simulink model "Lecture16_LSFIntegrator"  (R2020b)
settings: Solver=VariableStepAuto  StartTime=0.0  StopTime=10  RelTol=1e-3
values from neighbouring files (symbols this model uses):
  A = [0 1; -5 -2]    [Assignment4.m]    (also in Lecture14_LSF.m = [0 1; -1 -2]; Lecture15_DigitalLSF.m = [0 1; -1 -2]; Lecture16_LSFIntegrator.m = [0 1; -1 -2]; Lecture6_3PhaseCurrent.m = 20)
  B = [0; 1]    [Assignment4.m]    (also in Lecture14_LSF.m; Lecture15_DigitalLSF.m; Lecture16_LSFIntegrator.m; dSpaceLab.m = [0; 1/La])
  C = [5 0]    [Assignment4.m]    (also in Lecture14_LSF.m = [10 0]; Lecture15_DigitalLSF.m = [10 0]; Lecture16_LSFIntegrator.m = [10 0]; dSpaceLab.m = [1, 0])
  K12 = [K(1) K(2)]    [Assignment4.m]    (also in Lecture16_LSFIntegrator.m)
  Ki = 1/2    (= 0.5)    [Assignment3.m]    (also in Assignment4.m = -K(3); Lecture13_PolePlacement.m = 0.0125; Lecture16_LSFIntegrator.m = -K(3); Lecture4_DiscretePID.m = 0.8)
settings Model: Creator=sebastian  LastModifiedBy=sebastian

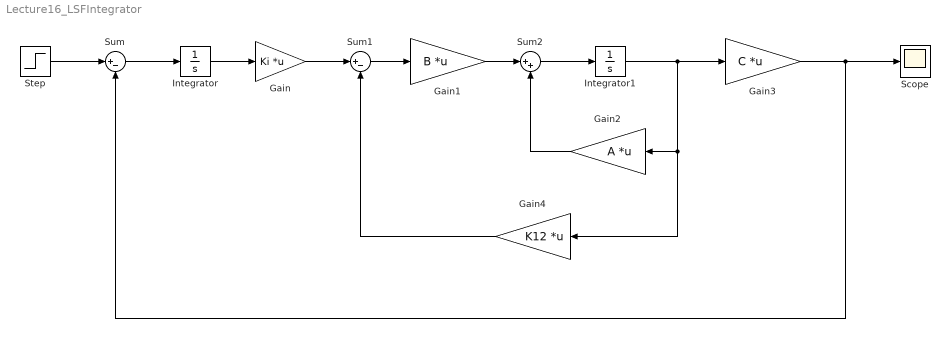
== system Lecture16_LSFIntegrator ==
  Gain : Gain  Gain=Ki  Multiplication=Matrix(K*u)
  Gain1 : Gain  Gain=B  Multiplication=Matrix(K*u)
  Gain2 : Gain  Gain=A  Multiplication=Matrix(K*u)
  Gain3 : Gain  Gain=C  Multiplication=Matrix(K*u)
  Gain4 : Gain  Gain=K12  Multiplication=Matrix(K*u)
  Integrator : Integrator
  Integrator1 : Integrator
  Scope : Scope
  Step : Step  SampleTime=0
  Sum : Sum  Inputs=|+-
  Sum1 : Sum  Inputs=|+-
  Sum2 : Sum  Inputs=|++
  wires:
  Step/1 -> Sum/1
  Sum/1 -> Integrator/1
  Integrator/1 -> Gain/1
  Gain/1 -> Sum1/1
  Sum1/1 -> Gain1/1
  Gain1/1 -> Sum2/1
  Gain2/1 -> Sum2/2
  Sum2/1 -> Integrator1/1
  Integrator1/1 -> Gain4/1, Gain2/1, Gain3/1
  Gain3/1 -> Sum/2, Scope/1
  Gain4/1 -> Sum1/2
